simulink model "Xplane Control Interface"  (R2024b)
settings: Solver=VariableStepAuto  StartTime=0.0  StopTime=inf  RelTol=1e-3
libraries: instrumentseriallib x2, etargetslib x2, sldrtlib x2, dspnetwork x2
settings Model: PacingRate=10  Creator=정예린  LastModifiedBy=banana99ou
settings RTWCC: GPUComputeCapability=3.5

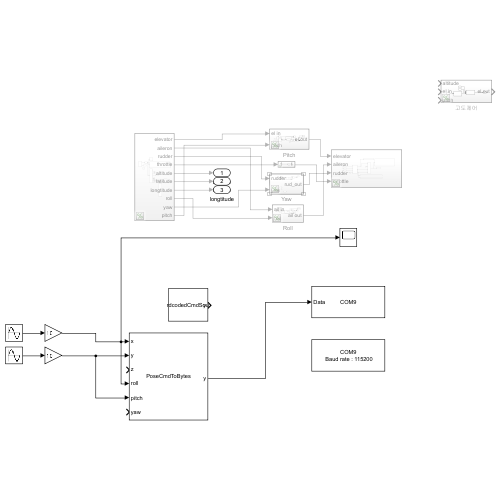
[thumbnail: Simulink's stored preview of the top-level diagram]
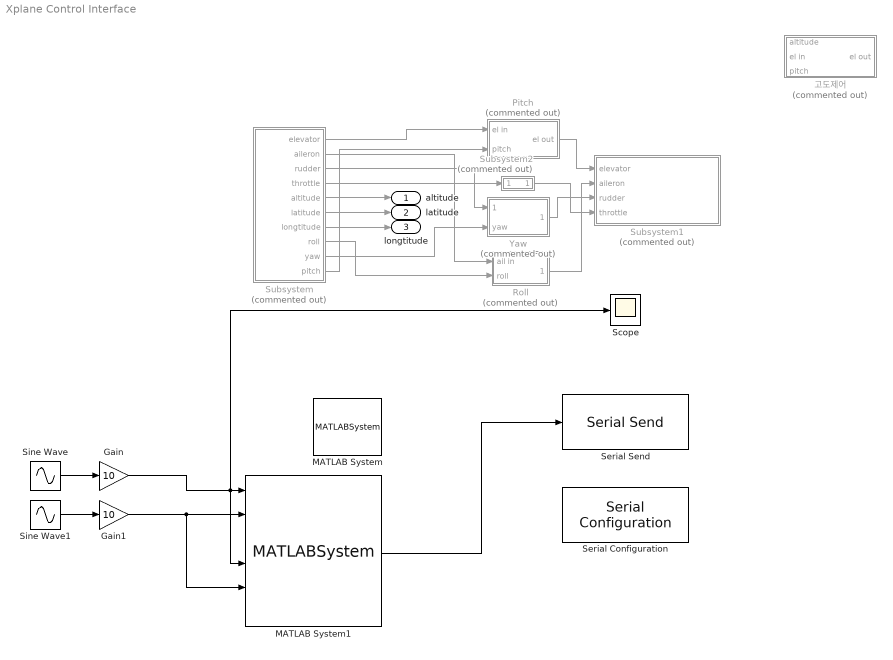
== system Xplane Control Interface ==
  Gain : Gain  Gain=10
  Gain1 : Gain  Gain=10
  MATLAB System : MATLABSystem  System=HardcodedCmdSource  Cmd=0 0 0 0 0 0  SimulateUsing=Code generation
      mask Type: HardcodedCmdSource
      mask Display:
      | disp('HardcodedCmdSource');
      | port_label('output',1,'y');
  MATLAB System1 : MATLABSystem  System=PoseCmdToBytes  Precision=3  MaxLen=128  PadByte=10  SimulateUsing=Code generation
      mask Type: PoseCmdToBytes
      mask Display:
      | disp('PoseCmdToBytes');
      | port_label('input',1,'x');
      | port_label('input',2,'y');
      | port_label('input',3,'z');
      | port_label('input',4,'roll');
      | port_label('input',5,'pitch');
      | port_label('input',6,'yaw');
      | port_label('output',1,'y');
  Pitch : Subsystem  Commented=on
  Roll : Subsystem  Commented=on
  Scope : Scope
  Serial Configuration : instrumentseriallib/Serial Configuration  Priority=-200000  PortSel=COM9  Port=COM9  ComPort=COM9  BaudRate=115200  DataBits=8  Parity=none  StopBits=1  ByteOrder=little-endian  FlowControl=none  Timeout=10  SimulateUsing=Interpreted execution  BlockInModel=on  aMode=1
  Serial Send : instrumentseriallib/Serial Send  Priority=1  PortSel=COM9  Port=COM9  ComPort=COM9  Header=[]  Terminator=<none>  CustomTerminator=[]  EnableBlockingMode=on  SimulateUsing=Interpreted execution  BlockInModel=on  aMode=1
  Sine Wave : Sin  Frequency=0.25  SampleTime=0
  Sine Wave1 : Sin  Frequency=0.25  Phase=1.5708  SampleTime=0
  Subsystem : Subsystem  Commented=on
  Subsystem1 : Subsystem  Commented=on
  Subsystem2 : Subsystem  Commented=on
  Yaw : Subsystem  Commented=on
  고도제어 : Subsystem  Commented=on
  altitude : Outport
  latitude : Outport  Port=2
  longtitude : Outport  Port=3
  wires:
  Subsystem/5(altitude) -> altitude/1
  Subsystem/6(latitude) -> latitude/1
  Subsystem/7(longtitude) -> longtitude/1
  Subsystem/9(yaw) -> Yaw/2(yaw)
  Subsystem/3(rudder) -> Yaw/1(rudder)
  Yaw/1(rud_out) -> Subsystem1/3(rudder)
  Subsystem/4(throttle) -> Subsystem2/1(In1)
  Subsystem2/1(Out1) -> Subsystem1/4(throttle)
  Subsystem/8(roll) -> Roll/2(roll)
  Subsystem/2(aileron) -> Roll/1(ail in)
  Roll/1(ail out) -> Subsystem1/2(aileron)
  Pitch/1(el out) -> Subsystem1/1(elevator)
  Subsystem/1(elevator) -> Pitch/1(el in)
  Subsystem/10(pitch) -> Pitch/2(pitch)
  MATLAB System1/1 -> Serial Send/1
  Sine Wave/1 -> Gain/1
  Sine Wave1/1 -> Gain1/1
  Gain1/1 -> MATLAB System1/2, MATLAB System1/5
  Gain/1 -> Scope/1, MATLAB System1/1, MATLAB System1/4

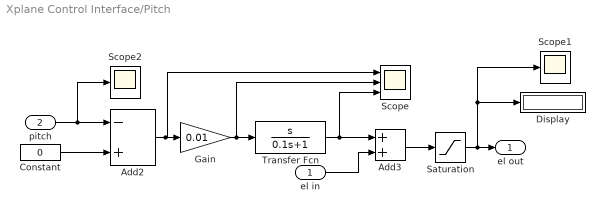
== system Xplane Control Interface/Pitch ==
  el in : Inport
  pitch : Inport  Port=2
  Add2 : Sum  Inputs=-+
  Add3 : Sum
  Constant : Constant  Value=0
  Display : Display
  Gain : Gain  Gain=0.01
  Saturation : Saturate  UpperLimit=1  LowerLimit=-1
  Scope : Scope  NumInputPorts=3
  Scope1 : Scope
  Scope2 : Scope
  Transfer Fcn : TransferFcn  Numerator=[1 0]  Denominator=[0.1 1]
  el out : Outport
  wires:
  el in/1 -> Add3/2
  Add3/1 -> Saturation/1
  Saturation/1 -> Scope1/1, Display/1, el out/1
  Gain/1 -> Scope/2, Transfer Fcn/1
  Add2/1 -> Scope/1, Gain/1
  Transfer Fcn/1 -> Scope/3, Add3/1
  Constant/1 -> Add2/2
  pitch/1 -> Scope2/1, Add2/1

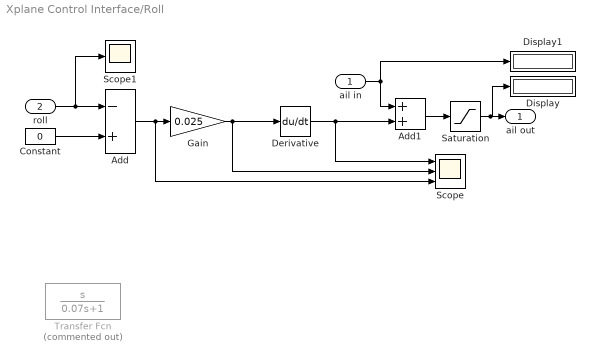
== system Xplane Control Interface/Roll ==
  ail in : Inport
  roll : Inport  Port=2
  Add : Sum  Inputs=-+
  Add1 : Sum
  Constant : Constant  Value=0
  Derivative : Derivative  CoefficientInTFapproximation=0.07
  Display : Display
  Display1 : Display
  Gain : Gain  Gain=0.025
  Saturation : Saturate  UpperLimit=1  LowerLimit=-1
  Scope : Scope  NumInputPorts=3
  Scope1 : Scope
  Transfer Fcn : TransferFcn  Commented=on  Numerator=[1 0]  Denominator=[0.07 1]
  ail out : Outport
  wires:
  Constant/1 -> Add/2
  Add/1 -> Scope/3, Gain/1
  Add1/1 -> Saturation/1
  ail in/1 -> Add1/1, Display1/1
  Saturation/1 -> ail out/1, Display/1
  roll/1 -> Scope1/1, Add/1
  Gain/1 -> Derivative/1, Scope/2
  Derivative/1 -> Scope/1, Add1/2

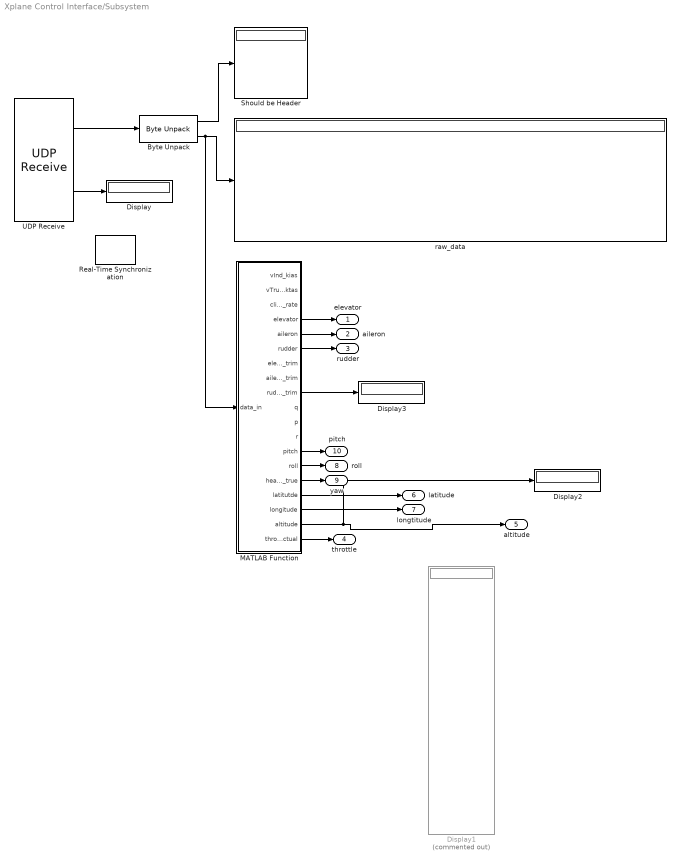
== system Xplane Control Interface/Subsystem ==
  Byte Unpack : etargetslib/Byte Unpack  dimensions={5,[9,8]}  datatypes={'uint8','single'}  byteAlign=1
  Display : Display
  Display1 : Display  Commented=on
  Display2 : Display
  Display3 : Display
  MATLAB Function : MATLAB Function  TreatAsAtomicUnit=on
  Real-Time Synchronization : sldrtlib/Real-Time Synchronization  SampleTime=0.1  MaxMissedTicks=10  ShowMissedTicks=off  YieldWhenWaiting=off
  Should be Header : Display
  UDP Receive : dspnetwork/UDP Receive  localURL='0.0.0.0'  localPort=49004  remoteURL='127.0.0.1'  remotePort=-1  recvBufferSize=8192  dims=293  signalDatatype=uint8  isComplex=off  isVarSize=off  showBlockingTime=off  blockingTime=0  sampletime=inf  blockPlatform=[]
  raw_data : Display
  elevator : Outport
  aileron : Outport  Port=2
  rudder : Outport  Port=3
  throttle : Outport  Port=4
  altitude : Outport  Port=5
  latitude : Outport  Port=6
  longtitude : Outport  Port=7
  roll : Outport  Port=8
  yaw : Outport  Port=9
  pitch : Outport  Port=10
  wires:
  Byte Unpack/1 -> Should be Header/1
  Byte Unpack/2 -> MATLAB Function/1(data_in), raw_data/1
  UDP Receive/2 -> Display/1
  UDP Receive/1 -> Byte Unpack/1
  MATLAB Function/4(elevator) -> elevator/1
  MATLAB Function/5(aileron) -> aileron/1
  MATLAB Function/6(rudder) -> rudder/1
  MATLAB Function/18(altitude) -> altitude/1, Display2/1
  MATLAB Function/19(throttle_actual) -> throttle/1
  MATLAB Function/16(latitutde) -> latitude/1
  MATLAB Function/17(longitude) -> longtitude/1
  MATLAB Function/14(roll) -> roll/1
  MATLAB Function/15(heading_true) -> yaw/1
  MATLAB Function/9(rudder_trim) -> Display3/1
  MATLAB Function/13(pitch) -> pitch/1

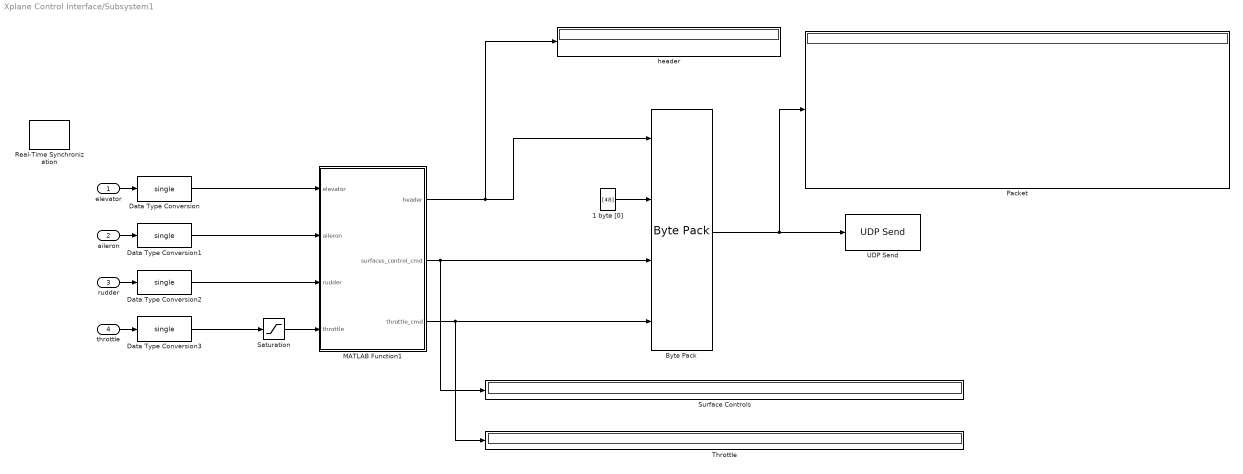
== system Xplane Control Interface/Subsystem1 ==
  elevator : Inport
  aileron : Inport  Port=2
  rudder : Inport  Port=3
  throttle : Inport  Port=4
  1 byte [0] : Constant  Value=[48]  OutDataTypeStr=uint8
  Byte Pack : etargetslib/Byte Pack  datatypes={'uint8','uint8','single','single'}  byteAlign=1
  Data Type Conversion{,1..3} (4 alike) : DataTypeConversion  OutDataTypeStr=single  SaturateOnIntegerOverflow=off  RndMeth=Floor
  MATLAB Function1 : MATLAB Function  TreatAsAtomicUnit=on
  Packet : Display
  Real-Time Synchronization : sldrtlib/Real-Time Synchronization  SampleTime=0.1  MaxMissedTicks=10  ShowMissedTicks=off  YieldWhenWaiting=off
  Saturation : Saturate  UpperLimit=1  LowerLimit=0
  Surface Controls : Display
  Throttle : Display
  UDP Send : dspnetwork/UDP Send  remoteURL='127.0.0.1'  remotePort=49000  localURL='0.0.0.0'  localPortSource=Automatically determine  localPort=-1  sendBufferSize=8192  sampletime=-1  blockPlatform=[]  separateLengthPort=0
  header : Display
  wires:
  MATLAB Function1/2(surfaces_control_cmd) -> Surface Controls/1, Byte Pack/3
  Saturation/1 -> MATLAB Function1/4(throttle)
  MATLAB Function1/1(header) -> Byte Pack/1, header/1
  1 byte [0]/1 -> Byte Pack/2
  Byte Pack/1 -> UDP Send/1, Packet/1
  MATLAB Function1/3(throttle_cmd) -> Throttle/1, Byte Pack/4
  elevator/1 -> Data Type Conversion/1
  aileron/1 -> Data Type Conversion1/1
  Data Type Conversion1/1 -> MATLAB Function1/2(aileron)
  rudder/1 -> Data Type Conversion2/1
  Data Type Conversion2/1 -> MATLAB Function1/3(rudder)
  throttle/1 -> Data Type Conversion3/1
  Data Type Conversion3/1 -> Saturation/1
  Data Type Conversion/1 -> MATLAB Function1/1(elevator)

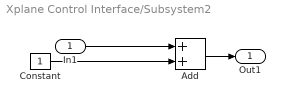
== system Xplane Control Interface/Subsystem2 ==
  In1 : Inport
  Add : Sum
  Constant : Constant
  Out1 : Outport
  wires:
  Constant/1 -> Add/2
  Add/1 -> Out1/1
  In1/1 -> Add/1

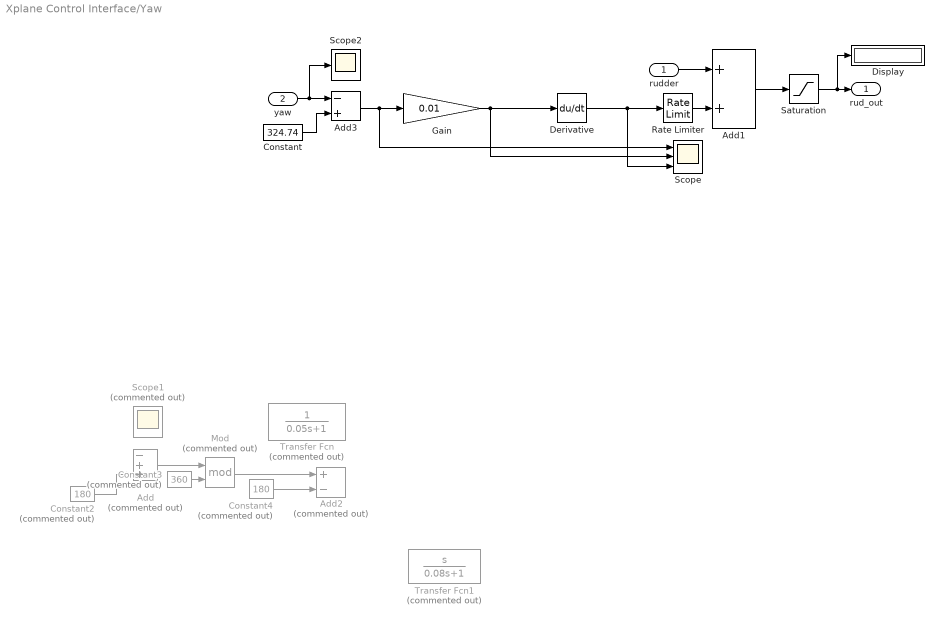
== system Xplane Control Interface/Yaw ==
  rudder : Inport
  yaw : Inport  Port=2
  Add : Sum  Commented=on  Inputs=-++
  Add1 : Sum
  Add2 : Sum  Commented=on  Inputs=+-
  Add3 : Sum  Inputs=-+
  Constant : Constant  Value=324.74
  Constant2 : Constant  Commented=on  Value=180
  Constant3 : Constant  Commented=on  Value=360
  Constant4 : Constant  Commented=on  Value=180
  Derivative : Derivative  CoefficientInTFapproximation=0.08
  Display : Display
  Gain : Gain  Gain=0.01
  Mod : Math  Commented=on  Operator=mod
  Rate Limiter : RateLimiter  RisingSlewLimit=0.5  FallingSlewLimit=-0.5  SampleTimeMode=inherited
  Saturation : Saturate  UpperLimit=1  LowerLimit=-1
  Scope : Scope  NumInputPorts=3
  Scope1 : Scope  Commented=on
  Scope2 : Scope
  Transfer Fcn : TransferFcn  Commented=on  Denominator=[0.05 1]
  Transfer Fcn1 : TransferFcn  Commented=on  Numerator=[1 0]  Denominator=[0.08 1]
  rud_out : Outport
  wires:
  Add1/1 -> Saturation/1
  rudder/1 -> Add1/1
  Saturation/1 -> Display/1, rud_out/1
  Gain/1 -> Derivative/1, Scope/2
  Constant2/1 -> Add/3
  Add/1 -> Mod/1
  Constant3/1 -> Mod/2
  Mod/1 -> Add2/1
  Constant4/1 -> Add2/2
  Add3/1 -> Scope/1, Gain/1
  yaw/1 -> Scope2/1, Add3/1
  Constant/1 -> Add3/2
  Rate Limiter/1 -> Add1/2
  Derivative/1 -> Scope/3, Rate Limiter/1

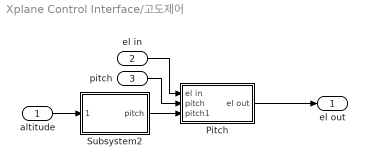
== system Xplane Control Interface/고도제어 ==
  altitude : Inport
  el in : Inport  Port=2
  pitch : Inport  Port=3
  Pitch : Subsystem
  Subsystem2 : Subsystem
  el out : Outport
  wires:
  Pitch/1(el out) -> el out/1
  Subsystem2/1(" pitch") -> Pitch/3(pitch1)
  altitude/1 -> Subsystem2/1(altitude)
  el in/1 -> Pitch/1(el in)
  pitch/1 -> Pitch/2(pitch)

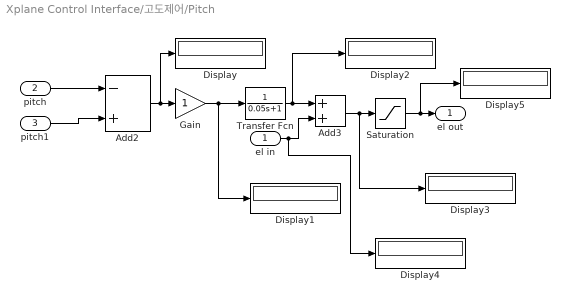
== system Xplane Control Interface/고도제어/Pitch ==
  el in : Inport
  pitch : Inport  Port=2
  pitch1 : Inport  Port=3
  Add2 : Sum  Inputs=-+
  Add3 : Sum
  Display{,1..5} (6 alike) : Display
  Gain : Gain
  Saturation : Saturate  UpperLimit=1  LowerLimit=-1
  Transfer Fcn : TransferFcn  Denominator=[0.05 1]
  el out : Outport
  wires:
  el in/1 -> Display4/1, Add3/2
  Add3/1 -> Display3/1, Saturation/1
  pitch1/1 -> Add2/2
  Saturation/1 -> Display5/1, el out/1
  Gain/1 -> Transfer Fcn/1, Display1/1
  Add2/1 -> Display/1, Gain/1
  Transfer Fcn/1 -> Display2/1, Add3/1
  pitch/1 -> Add2/1

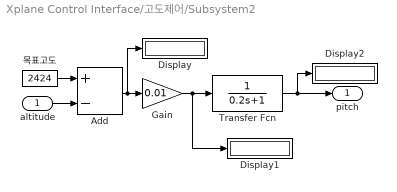
== system Xplane Control Interface/고도제어/Subsystem2 ==
  altitude : Inport
  Add : Sum  Inputs=+-
  Display : Display
  Display1 : Display
  Display2 : Display
  Gain : Gain  Gain=0.01
  Transfer Fcn : TransferFcn  Denominator=[0.2 1]
  목표고도 : Constant  Value=2424
  " pitch" : Outport
  wires:
  목표고도/1 -> Add/1
  altitude/1 -> Add/2
  Add/1 -> Display/1, Gain/1
  Gain/1 -> Transfer Fcn/1, Display1/1
  Transfer Fcn/1 -> Display2/1, " pitch"/1

== matlab function Xplane Control Interface/Subsystem1/MATLAB Function1 ==
  data: elevator input; header output uint8; surfaces_control_cmd output; aileron input single; rudder input single; throttle input; throttle_cmd output single
function [header,surfaces_control_cmd,throttle_cmd] = fcn(elevator, aileron, rudder, throttle) 
header =[uint8(68) uint8(65) uint8(84) uint8(65)];
No_Comand = single(-999);
 %Surface_header = typecast(uint8([uint8(8) uint8(0) uint8(0) uint8(0)]),'single')
surfaces_control_cmd = [1.1210388e-44 elevator aileron rudder No_Comand No_Comand No_Comand No_Comand No_Comand  ];
%Throttle_header = typecast(uint8([uint8(25) uint8(0) uint8(0) uint8(0)]),'single');
throttle_cmd = [3.503246160812043e-44 throttle No_Comand No_Comand No_Comand No_Comand No_Comand No_Comand No_Comand];
end

== matlab function Xplane Control Interface/Subsystem/MATLAB Function ==
  data: data_in input; vInd_kias output; vTrue_ktas output; climb_rate output; elevator output; aileron output; rudder output; elevator_trim output; aileron_trim output; rudder_trim output; q output; p output; r output; pitch output; roll output; heading_true output; latitutde output; longitude output; altitude output; throttle_actual output
function [vInd_kias,vTrue_ktas,...
    climb_rate,...
    elevator,aileron,rudder,...
    elevator_trim,aileron_trim,rudder_trim,...
    q,p,r,...
    pitch, roll, heading_true,...
    latitutde, longitude, altitude,...
    throttle_actual] = decoder(data_in)
 vInd_kias = data_in(2,1);
 vTrue_ktas = data_in(4,1);
 climb_rate = data_in(4,2);
 elevator = data_in(2,6);
 aileron = data_in(3,6);
 rudder= data_in(4,6);
 elevator_trim= data_in(2,7);
 aileron_trim= data_in(3,7);
 rudder_trim= data_in(4,7);
 q= data_in(2,5);
 p= data_in(3,5);
 r= data_in(4,5);
 pitch= data_in(2,3);
 roll= data_in(3,3);
 heading_true= data_in(4,3);
 latitutde= data_in(2,4);
 longitude= data_in(3,4);
 altitude= data_in(7,4);
 throttle_actual = data_in(2,8);
end
